simulink model "MyControl"  (R2017b)
settings: Solver=VariableStepAuto  StartTime=0.0  StopTime=35  RelTol=1e-3
libraries: xbsIndex_r4 x26
settings Model: Creator=manoh  LastModifiedBy=manoh

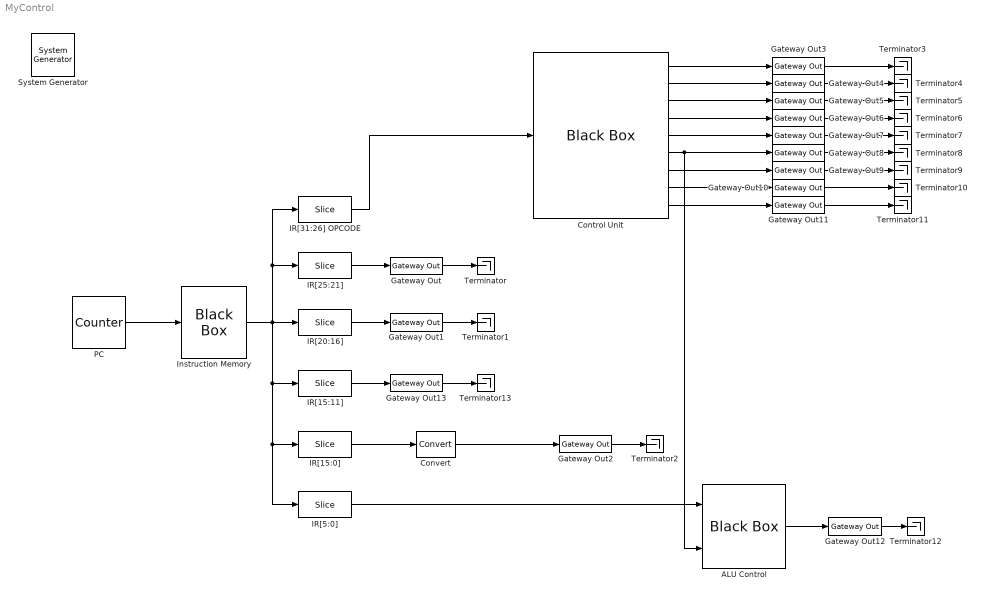
== system MyControl ==
  " System Generator" : xbsIndex_r4/ System Generator  Tag=genX  xilinxfamily=kintex7  part=xc7k325t  speed=-3  package=fbg676  synthesis_tool=Vivado  clock_wrapper=Clock Enables  directory=./netlist  proj_type=Vivado  Synth_file=Vivado Synthesis Defaults  Impl_file=Vivado Implementation Defaults  testbench=off  simulink_period=2  sysclk_period=10  dcm_input_clock_period=10  incr_netlist=off  trim_vbits=Everywhere in SubSystem  dbl_ovrd=According to Block Masks  core_generation=According to Block Masks  run_coregen=off  deprecated_control=off  eval_field=0  block_type=sysgen
  ALU Control : xbsIndex_r4/Black Box  init_code=ALUControl_config  sim_method=ISE Simulator  verbose=off  block_type=blackbox2
  Control Unit : xbsIndex_r4/Black Box  init_code=ControlUnit_config  sim_method=ISE Simulator  verbose=off  block_type=blackbox2
  Convert : xbsIndex_r4/Convert  gui_display_data_type=Fixed-point  arith_type="Signed  (2's comp)"  n_bits=32  bin_pt=0  float_type=Single  exp_bits=8  fraction_bits=24  quantization=Truncate  overflow=Wrap  en=off  latency=0  pipeline=off  dbl_ovrd=off  block_type=convert
  Gateway Out{,1..13} (14 alike) : xbsIndex_r4/Gateway Out  inherit_from_input=off  hdl_port=on  rows=1  columns=1  UseAsDAC=off  DACChannel='1'  interface=None  automatic_assignment=on  address_offset=hex2dec('00')  intf_name=''  intf_description=''  timing_constraint=None  locs_specified=off  LOCs={}  io_standard={}  block_type=gatewayout
  IR[15:0] : xbsIndex_r4/Slice  nbits=16  boolean_output=off  mode=Lower Bit Location + Width  bit1=-21  base1=MSB of Input  bit0=0  base0=LSB of Input  dbl_ovrd=off  block_type=slice
  IR[15:11] : xbsIndex_r4/Slice  nbits=5  boolean_output=off  mode=Upper Bit Location + Width  bit1=-16  base1=MSB of Input  bit0=0  base0=LSB of Input  dbl_ovrd=off  block_type=slice
  IR[20:16] : xbsIndex_r4/Slice  nbits=5  boolean_output=off  mode=Upper Bit Location + Width  bit1=-11  base1=MSB of Input  bit0=0  base0=LSB of Input  dbl_ovrd=off  block_type=slice
  IR[25:21] : xbsIndex_r4/Slice  nbits=5  boolean_output=off  mode=Upper Bit Location + Width  bit1=-6  base1=MSB of Input  bit0=0  base0=LSB of Input  dbl_ovrd=off  block_type=slice
  IR[31:26] OPCODE : xbsIndex_r4/Slice  nbits=6  boolean_output=off  mode=Upper Bit Location + Width  bit1=0  base1=MSB of Input  bit0=0  base0=LSB of Input  dbl_ovrd=off  block_type=slice
  IR[5:0] : xbsIndex_r4/Slice  nbits=6  boolean_output=off  mode=Lower Bit Location + Width  bit1=-21  base1=MSB of Input  bit0=0  base0=LSB of Input  dbl_ovrd=off  block_type=slice
  Instruction Memory : xbsIndex_r4/Black Box  init_code=InstructionMemory_config  sim_method=ISE Simulator  verbose=off  block_type=blackbox2
  PC : xbsIndex_r4/Counter  cnt_type=Free Running  cnt_to=Inf  operation=Up  start_count=0  cnt_by_val=4  arith_type=Unsigned  n_bits=32  bin_pt=0  load_pin=off  rst=off  en=off  explicit_period=on  period=2  use_behavioral_HDL=off  implementation=Fabric  dbl_ovrd=off  block_type=counter
  Terminator{,1..13} (14 alike) : Terminator
  wires:
  PC/1 -> Instruction Memory/1
  IR[15:0]/1 -> Convert/1
  IR[20:16]/1 -> Gateway Out1/1
  IR[31:26] OPCODE/1 -> Control Unit/1
  IR[25:21]/1 -> Gateway Out/1
  IR[5:0]/1 -> ALU Control/1
  Control Unit/6 -> Gateway Out8/1, ALU Control/2
  Gateway Out/1 -> Terminator/1
  Gateway Out1/1 -> Terminator1/1
  Gateway Out2/1 -> Terminator2/1
  Control Unit/1 -> Gateway Out3/1
  Control Unit/2 -> Gateway Out4/1
  Control Unit/3 -> Gateway Out5/1
  Control Unit/4 -> Gateway Out6/1
  Control Unit/5 -> Gateway Out7/1
  Control Unit/7 -> Gateway Out9/1
  Control Unit/8 -> Gateway Out10/1
  Control Unit/9 -> Gateway Out11/1
  ALU Control/1 -> Gateway Out12/1
  Gateway Out3/1 -> Terminator3/1
  Gateway Out4/1 -> Terminator4/1
  Gateway Out5/1 -> Terminator5/1
  Gateway Out6/1 -> Terminator6/1
  Gateway Out7/1 -> Terminator7/1
  Gateway Out8/1 -> Terminator8/1
  Gateway Out9/1 -> Terminator9/1
  Gateway Out10/1 -> Terminator10/1
  Gateway Out11/1 -> Terminator11/1
  Gateway Out12/1 -> Terminator12/1
  Gateway Out13/1 -> Terminator13/1
  IR[15:11]/1 -> Gateway Out13/1
  Convert/1 -> Gateway Out2/1
  Instruction Memory/1 -> IR[25:21]/1, IR[31:26] OPCODE/1, IR[15:0]/1, IR[5:0]/1, IR[15:11]/1, IR[20:16]/1
